simulink model "chap14_4"  (Simulink 7.5)
settings: Solver=FixedStepDiscrete  StartTime=0.0  StopTime=0.0  RelTol=1e-3
undefined symbols (not defined in the file): gray, Rec, SDTV
libraries: vipconversions x2, vipsnks x2, vipsrcs x1
settings Model: Creator=Administrator  LastModifiedBy=Administrator

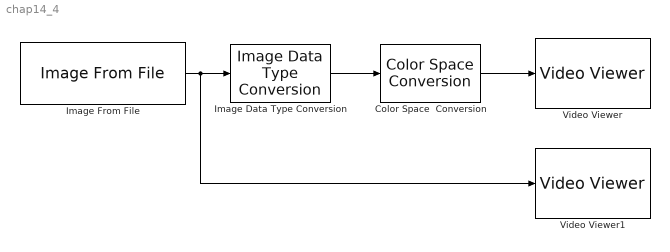
== system chap14_4 ==
  Color Space  Conversion : vipconversions/Color Space  Conversion  conversion=Obsolete  conversionActive=R'G'B' to HSV  wp_str=D65  rec=Rec. 601 (SDTV)  sys=1125/60/2:1  imagePorts=One multidimensional signal
  Image Data Type Conversion : vipconversions/Image Data Type Conversion  outDT=double  isSigned=on  wordLen=16  numFracBits=0
  Image From File : vipsrcs/Image From File  Tag=vipblks_nd  DialogController=vipDDGCreate  DialogControllerArgs=DataTag0  SystemSampleTime=-1  FileName=D:\Program Files\MATLAB\R2010a\toolbox\images\imdemos\pears.png  imagePorts=One multidimensional signal  Ts=inf  ImageDataType=Inherit from input image  Signed=on  WordLength=16  sdImageDataType=uint(8)  FractionLengthMode=User-defined  FractionLength=15  OutPortLabels=R|G|B
  Video Viewer : vipsnks/Video Viewer  DialogControllerArgs=DataTag2  inputType=Obsolete7b  imagePorts=One multidimensional signal  useColorMap=off  colormapValue=gray(256)  specRange=off  minInputVal=0  maxInputVal=255  FigPos=[180 612 410 300]  AxisZoom=on  trueSizedOnce=off  OpenAtMdlStart=on
  Video Viewer1 : vipsnks/Video Viewer  DialogControllerArgs=DataTag4  inputType=Obsolete7b  imagePorts=One multidimensional signal  useColorMap=off  colormapValue=gray(256)  specRange=off  minInputVal=0  maxInputVal=255  FigPos=[133 602 410 300]  AxisZoom=on  trueSizedOnce=off  OpenAtMdlStart=on
  wires:
  Color Space  Conversion/1 -> Video Viewer/1
  Image From File/1 -> Image Data Type Conversion/1, Video Viewer1/1
  Image Data Type Conversion/1 -> Color Space  Conversion/1
